simulink model "InkrementalisSimulation"  (R2013b)
settings: Solver=FixedStepDiscrete  SolverMode=SingleTasking  StartTime=0.0  StopTime=190  FixedStep=0.1  RelTol=1e-3
libraries: xbsIndex_r4 x6, simulink x2
settings Model: Creator=laca  LastModifiedBy=laca

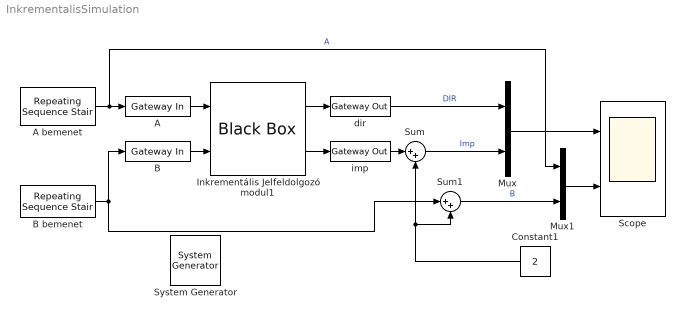
== system InkrementalisSimulation ==
  " System Generator" : xbsIndex_r4/ System Generator  Tag=genX  xilinxfamily=spartan3e  part=xc3s500e  speed=-4  package=pq208  synthesis_tool=XST  clock_wrapper=Clock Enables  directory=./netlist  proj_type=Project Navigator  Synth_file=XST Defaults  Impl_file=ISE Defaults  testbench=off  simulink_period=1  sysclk_period=20  dcm_input_clock_period=10  incr_netlist=off  trim_vbits=Everywhere in SubSystem  dbl_ovrd=According to Block Masks  core_generation=According to Block Masks  run_coregen=off  deprecated_control=off  eval_field=0  block_type=sysgen
  A : xbsIndex_r4/Gateway In  gui_display_data_type=Boolean  arith_type=Boolean  n_bits=16  bin_pt=14  preci_type=Single  exp_width=8  frac_width=24  quantization="Round  (unbiased: +/- Inf)"  overflow=Saturate  period=1  dbl_ovrd=off  timing_constraint=None  locs_specified=off  LOCs={}  UseAsADC=off  ADCChannel='1'  inherit_from_input=off  hdl_port=on  block_type=gatewayin
  A bemenet : simulink/Sources/Repeating Sequence Stair  OutValues="[ 0 0 1 1 1 1 1 0 0 0 0 0 1 1 1 1 1 0 0 0 0 0 1 1 1 1 1 0 0 0 0 0 1 1 1 1 1 0 0 0 1 1 1 1 1 0 0 0 0 0 1 1 1 1 1 0 0 0 0 0 1 1 1 1 1 0 0 0 0 0 1 1 1 1 1 0 0 0 0 0 0 0 0 1 1  0 0 0 0 0 0 0 0 1 1 0 0 0 0 0 0 0 0 1 1  0 0 0 0 0 0 0 0 1 1 0 0 0 0 0 0 0 0 0 0 0 0 0 0 0 0 0 0 0 0 0 0 0 0 0 0 0 0 0 0 0 0 0 0 0 0 0 0 0 0 0 0 0 0 0 0 1 1 0 0 0 0 0 0 0 0 1 1 0 0 0 0 0 0 0 0 1 1 0 0 0 0 ].'"  tsamp=1  OutMin=[]  OutMax=[]  OutDataTypeStr=double  OutputDataTypeScalingMode=double  OutDataType=fixdt(0,8)  ConRadixGroup=Best Precision: Vector-wise  OutScaling=2^-12
  B : xbsIndex_r4/Gateway In  gui_display_data_type=Boolean  arith_type=Boolean  n_bits=16  bin_pt=14  preci_type=Single  exp_width=8  frac_width=24  quantization="Round  (unbiased: +/- Inf)"  overflow=Saturate  period=1  dbl_ovrd=off  timing_constraint=None  locs_specified=off  LOCs={}  UseAsADC=off  ADCChannel='1'  inherit_from_input=off  hdl_port=on  block_type=gatewayin
  B bemenet : simulink/Sources/Repeating Sequence Stair  OutValues="[1 1 1 1 1 0 0 0 0 0 1 1 1 1 1 0 0 0 0 0 1 1 1 1 1 0 0 0 0 0 1 1 1 1 1 0 0 0 0 0 0 1 1 1 1 1 0 0 0 0 0 1 1 1 1 1 0 0 0 0 0 1 1 1 1 1 0 0 0 0 0 1 1 1 1 1 0 0 0  0 0 1 1 1 1 1 0 0 0  0 0 1 1 1 1 1 0 0 0  0 0 1 1 1 1 1 0 0 0  0 0 1 1 1 1 1 0 0 0  0 0 1 1 1 1 1 0 0 0  0 0 1 1 1 1 1 0 0 0 0 0 0 0 0 0 0 0 0 0 0 0 0 0 0 1 1 1 1 1 1 1 1 1 1 1 1 1 1 1 1 1 1 1 1 1 1 1 1 1 1 1 1 1 1].'"  tsamp=1  OutMin=[]  OutMax=[]  OutDataTypeStr=double  OutputDataTypeScalingMode=double  OutDataType=fixdt(0,8)  ConRadixGroup=Best Precision: Vector-wise  OutScaling=2^-12
  Constant1 : Constant  Value=2
  Inkrementális Jelfeldolgozó modul1 : xbsIndex_r4/Black Box  init_code=IncSensor_config  sim_method=ISE Simulator  verbose=off  block_type=blackbox2
  Mux : Mux  Inputs=2
  Mux1 : Mux  Inputs=2
  Scope : Scope  NumInputPorts=2
      settings: TickLabels=on  ShowLegends=on  YMin=-5~-5  YMax=5~5
  Sum : Sum  Inputs=|++
  Sum1 : Sum  Inputs=|++
  dir : xbsIndex_r4/Gateway Out  inherit_from_input=off  hdl_port=on  timing_constraint=None  locs_specified=off  LOCs={}  UseAsDAC=off  DACChannel='1'  block_type=gatewayout
  imp : xbsIndex_r4/Gateway Out  inherit_from_input=off  hdl_port=on  timing_constraint=None  locs_specified=off  LOCs={}  UseAsDAC=off  DACChannel='1'  block_type=gatewayout
  wires:
  A/1 -> Inkrementális Jelfeldolgozó modul1/1
  B/1 -> Inkrementális Jelfeldolgozó modul1/2
  Inkrementális Jelfeldolgozó modul1/1 -> dir/1
  Inkrementális Jelfeldolgozó modul1/2 -> imp/1
  Mux/1 -> Scope/1
  dir/1 -> Mux/1  "DIR"
  imp/1 -> Sum/1
  Sum/1 -> Mux/2  "Imp"
  B bemenet/1 -> B/1, Sum1/1
  A bemenet/1 -> Mux1/1, A/1  "A"
  Mux1/1 -> Scope/2
  Sum1/1 -> Mux1/2  "B"
  Constant1/1 -> Sum1/2, Sum/2
